simulink library "Constant_Environment"  (R2018b)
settings: Solver=VariableStepAuto  StartTime=0.0  StopTime=10.0  RelTol=1e-3
settings Model: Creator=Alexander Koch  LastModifiedBy=ga69qig
settings SFSimCC: SimUseLocalCustomCode=off
settings RTWCC: RTWUseLocalCustomCode=off
settings CodeAppCC: StateflowObjectComments=on

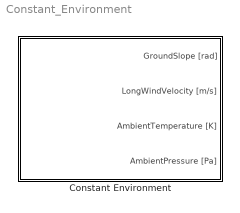
== system Constant_Environment ==
  Constant Environment : Subsystem  mask(SB){Ground_Slope=0, Long_Wind_Speed=0, Ambient_P=101325, Ambient_Temp=298.15, LocalSampleTime=-1}
      mask prompts: Ground_Slope "Ground Slope [rad]"; Long_Wind_Speed "Longitudinal Wind Velocity [m/s]"; Ambient_P "Ambient Pressure [Pa]"; Ambient_Temp "Ambient Temperature [K]"; LocalSampleTime "Local System Sample-Time [s]"
      mask help:
      | <Author> Tony Weiss based on Alexander Koch </Author>
      | <Date> 31/12/2017 </Date>
      | <Source>
      | [1] A. Koch, “Aufbau einer modularen Komponentenbibliothek für Gesamtfahrzeugsimulationen in Matlab/Simulink,” Technische Universität München, München, 2017
      | </Source>
      |
      | <Description>
      | Requires a ground slope, a longitudinal wind velocity, an ambient temperature and an ambient pressure and gives these constant values as signals. Ambient pressure is preset to 101325 Pa (standard pressure at sea level), ambient temperature is preset to 298.15 K.
      | </Description>
      mask init:
      | GlobalSampleTime = CalcGlobalSampleTime(LocalSampleTime);
      mask Help:
      | <Parameters>
      | Ground Slope [rad]
      | Longitudinal Wind Velocity [m/s]
      | Ambient Temperature [K]
      | Ambient Pressure [Pa]
      | Local System Sample-Time [s]
      | 	<Min> GlobalSampleTime </Min>
      | Global Sample-Time [s]
      | </Parameters>
      | 
      | <Inputs>
      | </Inputs>
      | 
      | <Outputs>
      | GroundSlope [rad]
      | LongWindVelocity [m/s]
      | AmbientTemperature [K]
      | AmbientPressure [Pa]
      | </Outputs>
      mask TypeOptions Ground_Slope: Const_Ground_Slope/Value
      mask TypeOptions Long_Wind_Speed: Const_Long_Wind_Velocity/Value
      mask TypeOptions Ambient_P: Const_Ambient_Pressure/Value
      mask TypeOptions Ambient_Temp: Const_Ambient_Temperature/Value
      mask TypeOptions LocalSampleTime: Const_Ambient_Pressure/SampleTime | Const_Ambient_Temperature/SampleTime | Const_Ground_Slope/SampleTime | Const_Long_Wind_Velocity/SampleTime
      mask DialogControl Container3 Prompt: Documentation:
      mask DialogControl Control2 Prompt: %<MaskHelp>
      mask DialogControl Container5 Prompt: Sample Time
      mask Display:
      | [picturexpos,pictureypos,picturewidth,pictureheight] = ...
      |     CalcBlockPicturePosition(gcb,1,0.01,0.1,10,100); % calculating picture position depending on Block size and minimum margin size
      | image('Constant_Environment.svg',[picturexpos pictureypos picturewidth pictureheight]) % plot picture to block

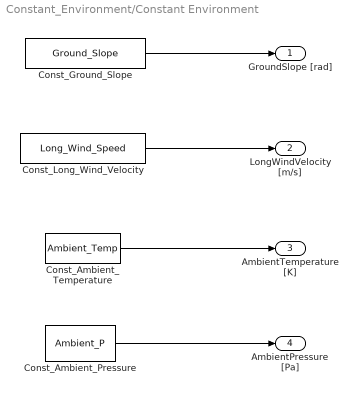
== system Constant_Environment/Constant Environment ==
  Const_Ambient_Pressure : Constant  Value=Ambient_P  SampleTime=LocalSampleTime
  Const_Ambient_Temperature : Constant  Value=Ambient_Temp  SampleTime=LocalSampleTime
  Const_Ground_Slope : Constant  Value=Ground_Slope  SampleTime=LocalSampleTime
  Const_Long_Wind_Velocity : Constant  Value=Long_Wind_Speed  SampleTime=LocalSampleTime
  GroundSlope [rad] : Outport  SampleTime=GlobalSampleTime
  LongWindVelocity [m/s] : Outport  Port=2  SampleTime=GlobalSampleTime
  AmbientTemperature [K] : Outport  Port=3  SampleTime=GlobalSampleTime
  AmbientPressure [Pa] : Outport  Port=4  SampleTime=GlobalSampleTime
  wires:
  Const_Long_Wind_Velocity/1 -> LongWindVelocity [m/s]/1
  Const_Ground_Slope/1 -> GroundSlope [rad]/1
  Const_Ambient_Temperature/1 -> AmbientTemperature [K]/1
  Const_Ambient_Pressure/1 -> AmbientPressure [Pa]/1
